simulink library "sadc_library_old"  (R2020b)
settings: Solver=VariableStepAuto  StartTime=0.0  StopTime=10.0  RelTol=1e-3
undefined symbols (not defined in the file or in its folder): magnitude
libraries: vrlib x4
settings Model: Creator=loren  LastModifiedBy=loren

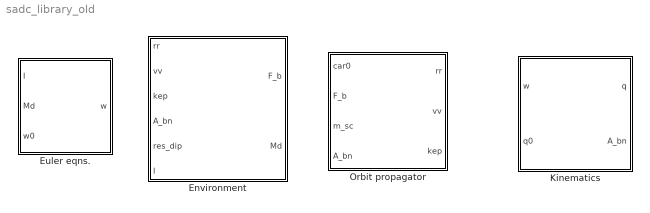
== system sadc_library_old ==
  Environment : Subsystem
  Euler eqns. : Subsystem
  Kinematics : Subsystem
  Orbit propagator : Subsystem

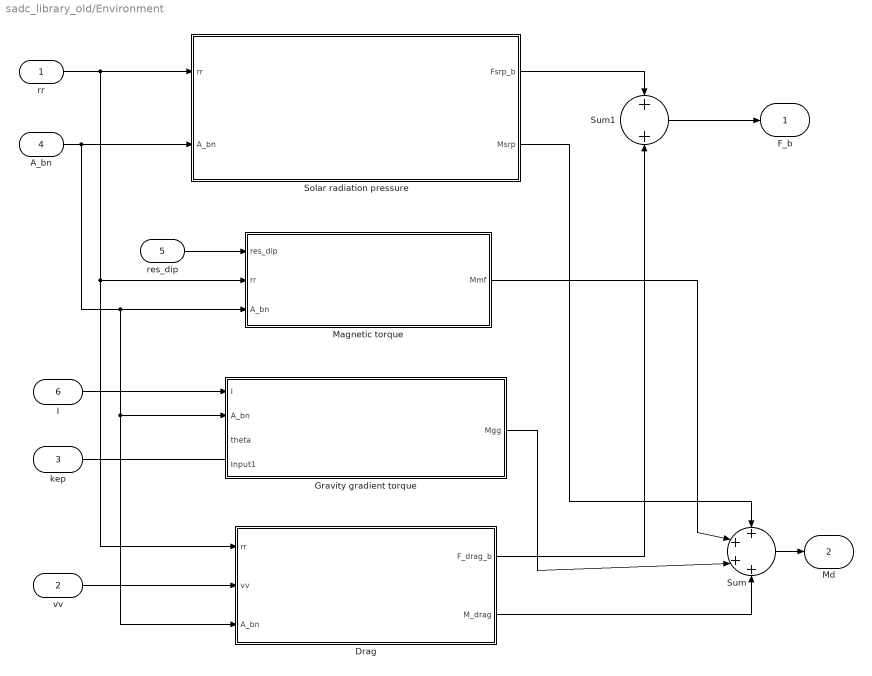
== system sadc_library_old/Environment ==
  rr : Inport
  vv : Inport  Port=2
  kep : Inport  Port=3
  A_bn : Inport  Port=4
  res_dip : Inport  Port=5
  I : Inport  Port=6
  Drag : Subsystem
  Gravity gradient torque : Subsystem
  Magnetic torque : Subsystem
  Solar radiation pressure : Subsystem
  Sum : Sum  Inputs=++++
  Sum1 : Sum
  F_b : Outport
  Md : Outport  Port=2
  wires:
  kep/1 -> ?
  Solar radiation pressure/1(Fsrp_b) -> Sum1/1
  Solar radiation pressure/2(Msrp) -> Sum/1
  A_bn/1 -> Drag/3(A_bn), Gravity gradient torque/2(A_bn), Magnetic torque/3(A_bn), Solar radiation pressure/2(A_bn)
  vv/1 -> Drag/2(vv)
  rr/1 -> Magnetic torque/2(rr), Drag/1(rr), Solar radiation pressure/1(rr)
  Gravity gradient torque/1(Mgg) -> Sum/3
  Drag/2(M_drag) -> Sum/4
  Drag/1(F_drag_b) -> Sum1/2
  I/1 -> Gravity gradient torque/1(I)
  res_dip/1 -> Magnetic torque/1(res_dip)
  Magnetic torque/1(Mmf) -> Sum/2
  Sum1/1 -> F_b/1
  Sum/1 -> Md/1

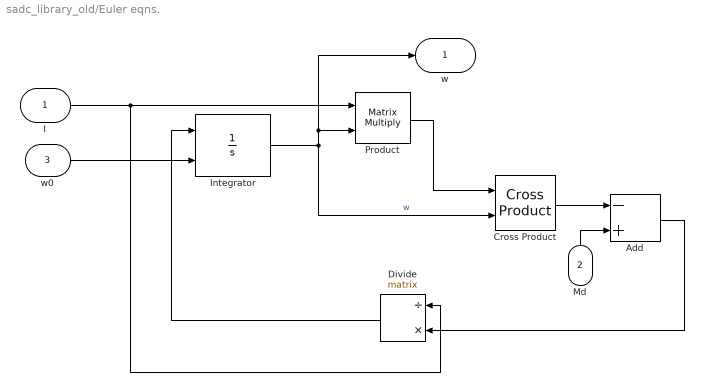
== system sadc_library_old/Euler eqns. ==
  I : Inport
  Md : Inport  Port=2
  w0 : Inport  Port=3
  Add : Sum  Inputs=-+
  Cross Product : vrlib/Utilities/Cross Product
  Divide : Product  Inputs=/*  Multiplication=Matrix(*)
  Integrator : Integrator  InitialConditionSource=external
  Product : Product  Multiplication=Matrix(*)
  w : Outport
  wires:
  I/1 -> Divide/1, Product/1
  w0/1 -> Integrator/2
  Integrator/1 -> Product/2, w/1, Cross Product/2  "w"
  Product/1 -> Cross Product/1
  Md/1 -> Add/2
  Cross Product/1 -> Add/1
  Add/1 -> Divide/2
  Divide/1 -> Integrator/1

== system sadc_library_old/Kinematics ==
  w : Inport
  q0 : Inport  Port=2
  DCM : Subsystem
  Quaternion integration : Subsystem
  q : Outport
  A_bn : Outport  Port=2
  wires:
  w/1 -> Quaternion integration/1(w)
  q0/1 -> Quaternion integration/2(q0)
  Quaternion integration/1(q) -> q/1, DCM/1(q)
  DCM/1(A_bn) -> A_bn/1

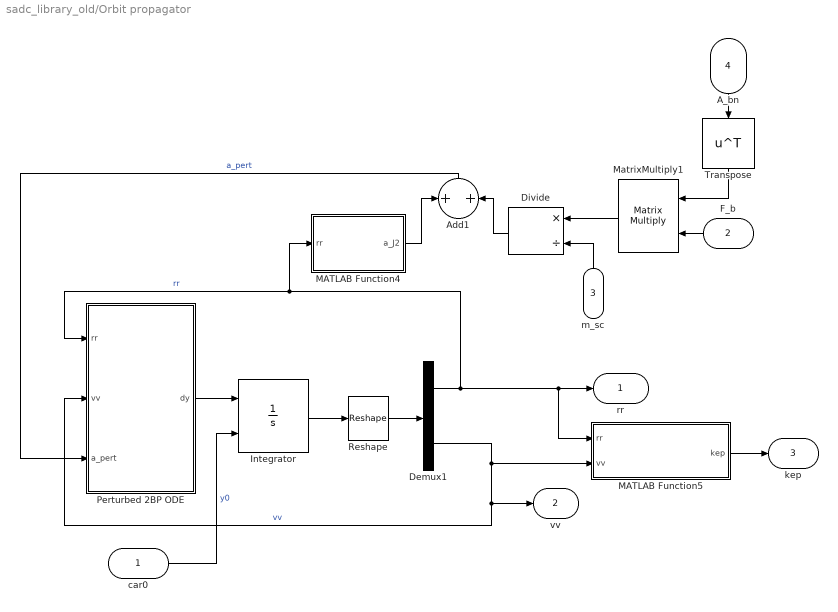
== system sadc_library_old/Orbit propagator ==
  car0 : Inport
  F_b : Inport  Port=2
  m_sc : Inport  Port=3
  A_bn : Inport  Port=4
  Add1 : Sum
  Demux1 : Demux  Outputs=[3,3]
  Divide : Product  Inputs=*/
  Integrator : Integrator  InitialConditionSource=external
  MATLAB Function4 : MATLAB Function  TreatAsAtomicUnit=on
  MATLAB Function5 : MATLAB Function  TreatAsAtomicUnit=on
  MatrixMultiply1 : Product  Multiplication=Matrix(*)
  Perturbed 2BP ODE : Subsystem
  Reshape : Reshape  OutputDimensionality=Column vector (2-D)
  Transpose : Math  Operator=transpose  SaturateOnIntegerOverflow=on
  rr : Outport
  vv : Outport  Port=2
  kep : Outport  Port=3
  wires:
  Integrator/1 -> Reshape/1
  Demux1/1 -> MATLAB Function5/1(rr), rr/1, MATLAB Function4/1(rr), Perturbed 2BP ODE/1(rr)  "rr"
  Perturbed 2BP ODE/1(dy) -> Integrator/1
  Demux1/2 -> vv/1, Perturbed 2BP ODE/2(vv), MATLAB Function5/2(vv)  "vv"
  car0/1 -> Integrator/2  "y0"
  Add1/1 -> Perturbed 2BP ODE/3(a_pert)  "a_pert"
  MATLAB Function4/1(a_J2) -> Add1/1
  F_b/1 -> MatrixMultiply1/2
  MatrixMultiply1/1 -> Divide/1
  m_sc/1 -> Divide/2
  Divide/1 -> Add1/2
  MATLAB Function5/1(kep) -> kep/1
  A_bn/1 -> Transpose/1
  Transpose/1 -> MatrixMultiply1/1
  Reshape/1 -> Demux1/1

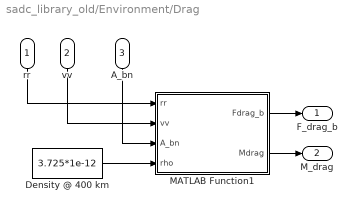
== system sadc_library_old/Environment/Drag ==
  rr : Inport
  vv : Inport  Port=2
  A_bn : Inport  Port=3
  Density @ 400 km : Constant  Value=3.725*1e-12
  MATLAB Function1 : MATLAB Function  TreatAsAtomicUnit=on
  F_drag_b : Outport
  M_drag : Outport  Port=2
  wires:
  rr/1 -> MATLAB Function1/1(rr)
  MATLAB Function1/1(Fdrag_b) -> F_drag_b/1
  MATLAB Function1/2(Mdrag) -> M_drag/1
  vv/1 -> MATLAB Function1/2(vv)
  A_bn/1 -> MATLAB Function1/3(A_bn)
  Density @ 400 km/1 -> MATLAB Function1/4(rho)

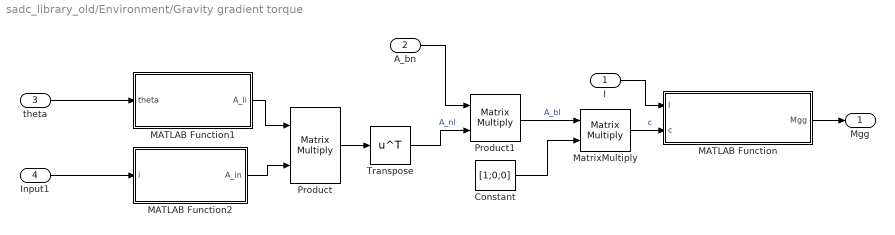
== system sadc_library_old/Environment/Gravity gradient torque ==
  I : Inport
  A_bn : Inport  Port=2
  theta : Inport  Port=3
  Input1 : Inport  Port=4
  Constant : Constant  Value=[1;0;0]
  MATLAB Function : MATLAB Function  TreatAsAtomicUnit=on
  MATLAB Function1 : MATLAB Function  TreatAsAtomicUnit=on
  MATLAB Function2 : MATLAB Function  TreatAsAtomicUnit=on
  MatrixMultiply : Product  Multiplication=Matrix(*)
  Product : Product  Multiplication=Matrix(*)
  Product1 : Product  Multiplication=Matrix(*)
  Transpose : Math  Operator=transpose  SaturateOnIntegerOverflow=on
  Mgg : Outport
  wires:
  I/1 -> MATLAB Function/1(I)
  Product/1 -> Transpose/1
  Transpose/1 -> Product1/2  "A_nl"
  Product1/1 -> MatrixMultiply/1  "A_bl"
  A_bn/1 -> Product1/1
  Constant/1 -> MatrixMultiply/2
  MatrixMultiply/1 -> MATLAB Function/2(c)  "c"
  MATLAB Function/1(Mgg) -> Mgg/1
  MATLAB Function2/1(A_in) -> Product/2
  MATLAB Function1/1(A_li) -> Product/1
  theta/1 -> MATLAB Function1/1(theta)
  Input1/1 -> MATLAB Function2/1(i)

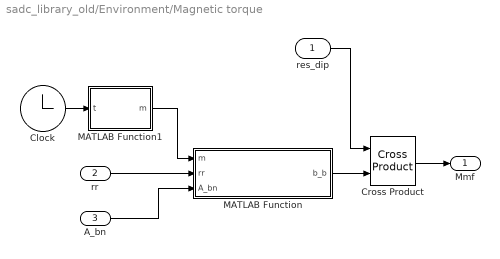
== system sadc_library_old/Environment/Magnetic torque ==
  res_dip : Inport
  rr : Inport  Port=2
  A_bn : Inport  Port=3
  Clock : Clock
  Cross Product : vrlib/Utilities/Cross Product
  MATLAB Function : MATLAB Function  TreatAsAtomicUnit=on
  MATLAB Function1 : MATLAB Function  TreatAsAtomicUnit=on
  Mmf : Outport
  wires:
  Cross Product/1 -> Mmf/1
  Clock/1 -> MATLAB Function1/1(t)
  rr/1 -> MATLAB Function/2(rr)
  A_bn/1 -> MATLAB Function/3(A_bn)
  res_dip/1 -> Cross Product/1
  MATLAB Function/1(b_b) -> Cross Product/2
  MATLAB Function1/1(m) -> MATLAB Function/1(m)

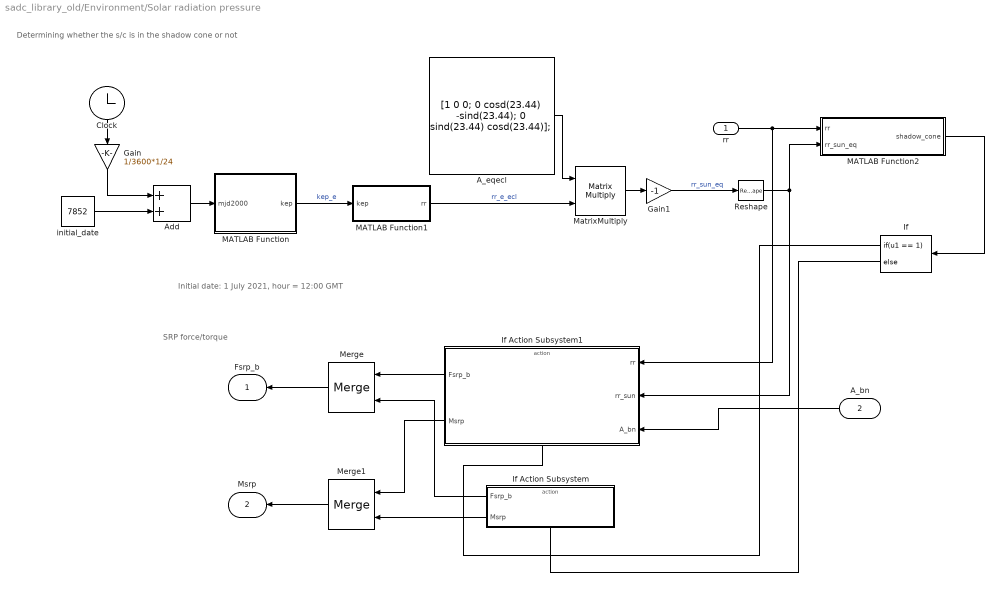
== system sadc_library_old/Environment/Solar radiation pressure ==
  note: SRP force/torque
  note: Initial date: 1 July 2021,
      | hour = 12:00 GMT
  note: Determining whether the s/c is in the shadow cone or not
  rr : Inport
  A_bn : Inport  Port=2
  A_eqecl : Constant  Value=|
      | [1   0   0;
      |     0  cosd(23.44)  -sind(23.44);
      |     0  sind(23.44)  cosd(23.44)];
  Add : Sum
  Clock : Clock
  Gain : Gain  Gain=1/3600*1/24
  Gain1 : Gain  Gain=-1
  If : If  IfExpression=u1 == 1
  If Action Subsystem : Subsystem  TreatAsAtomicUnit=on
  If Action Subsystem1 : Subsystem  TreatAsAtomicUnit=on
  MATLAB Function : MATLAB Function  TreatAsAtomicUnit=on
  MATLAB Function1 : MATLAB Function  TreatAsAtomicUnit=on
  MATLAB Function2 : MATLAB Function  TreatAsAtomicUnit=on
  MatrixMultiply : Product  Multiplication=Matrix(*)
  Merge : Merge
  Merge1 : Merge
  Reshape : Reshape  OutputDimensionality=Column vector (2-D)
  initial_date : Constant  Value=7852
  Fsrp_b : Outport
  Msrp : Outport  Port=2
  wires:
  initial_date/1 -> Add/2
  Clock/1 -> Gain/1
  Add/1 -> MATLAB Function/1(mjd2000)
  Gain/1 -> Add/1
  MatrixMultiply/1 -> Gain1/1
  MATLAB Function1/1(rr) -> MatrixMultiply/2  "rr_e_ecl"
  MATLAB Function/1(kep) -> MATLAB Function1/1(kep)  "kep_e"
  Gain1/1 -> Reshape/1  "rr_sun_eq"
  MATLAB Function2/1(shadow_cone) -> If/1
  If/2 -> If Action Subsystem/Action
  If/1 -> If Action Subsystem1/Action
  If Action Subsystem/1(Fsrp_b) -> Merge/2
  If Action Subsystem/2(Msrp) -> Merge1/2
  rr/1 -> MATLAB Function2/1(rr), If Action Subsystem1/1(rr)
  Merge/1 -> Fsrp_b/1
  Merge1/1 -> Msrp/1
  If Action Subsystem1/1(Fsrp_b) -> Merge/1
  If Action Subsystem1/2(Msrp) -> Merge1/1
  A_bn/1 -> If Action Subsystem1/3(A_bn)
  A_eqecl/1 -> MatrixMultiply/1
  Reshape/1 -> MATLAB Function2/2(rr_sun_eq), If Action Subsystem1/2(rr_sun)

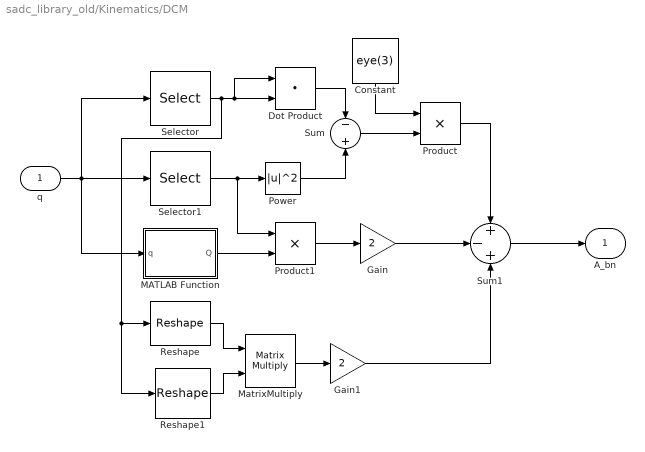
== system sadc_library_old/Kinematics/DCM ==
  q : Inport
  Constant : Constant  Value=eye(3)
  Dot Product : DotProduct  InputSameDT=on  OutDataTypeStr=Inherit: Inherit via internal rule
  Gain : Gain  Gain=2
  Gain1 : Gain  Gain=2
  MATLAB Function : MATLAB Function  TreatAsAtomicUnit=on
  MatrixMultiply : Product  Multiplication=Matrix(*)
  Power : Math  Operator=magnitude^2  SaturateOnIntegerOverflow=on
  Product : Product
  Product1 : Product
  Reshape : Reshape  OutputDimensionality=Column vector (2-D)
  Reshape1 : Reshape  OutputDimensionality=Row vector (2-D)
  Selector : Selector  InputPortWidth=4  IndexOptions=Index vector (dialog)  Indices=[1 2 3]  OutputSizes=1
  Selector1 : Selector  InputPortWidth=4  IndexOptions=Index vector (dialog)  Indices=[4]  OutputSizes=1
  Sum : Sum  Inputs=-+
  Sum1 : Sum  Inputs=+-+
  A_bn : Outport
  wires:
  q/1 -> MATLAB Function/1(q), Selector1/1, Selector/1
  Selector/1 -> Reshape1/1, Reshape/1, Dot Product/2, Dot Product/1
  Selector1/1 -> Product1/1, Power/1
  Power/1 -> Sum/2
  Dot Product/1 -> Sum/1
  Constant/1 -> Product/1
  Sum/1 -> Product/2
  MATLAB Function/1(Q) -> Product1/2
  Product1/1 -> Gain/1
  Reshape/1 -> MatrixMultiply/1
  Reshape1/1 -> MatrixMultiply/2
  MatrixMultiply/1 -> Gain1/1
  Product/1 -> Sum1/1
  Gain/1 -> Sum1/2
  Gain1/1 -> Sum1/3
  Sum1/1 -> A_bn/1

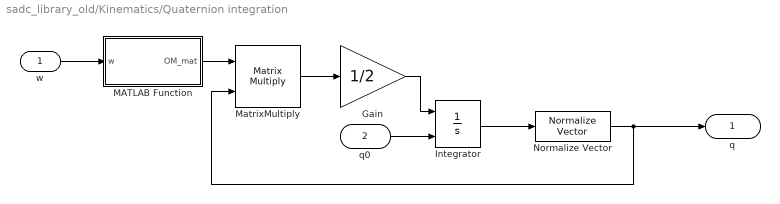
== system sadc_library_old/Kinematics/Quaternion integration ==
  w : Inport
  q0 : Inport  Port=2
  Gain : Gain  Gain=1/2
  Integrator : Integrator  InitialConditionSource=external
  MATLAB Function : MATLAB Function  TreatAsAtomicUnit=on
  MatrixMultiply : Product  Multiplication=Matrix(*)
  Normalize Vector : vrlib/Utilities/Normalize Vector  maxzero=0
  q : Outport
  wires:
  Integrator/1 -> Normalize Vector/1
  w/1 -> MATLAB Function/1(w)
  Normalize Vector/1 -> q/1, MatrixMultiply/2
  q0/1 -> Integrator/2
  MATLAB Function/1(OM_mat) -> MatrixMultiply/1
  MatrixMultiply/1 -> Gain/1
  Gain/1 -> Integrator/1

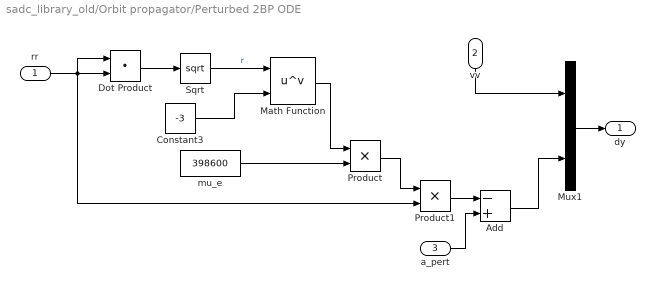
== system sadc_library_old/Orbit propagator/Perturbed 2BP ODE ==
  rr : Inport
  vv : Inport  Port=2
  a_pert : Inport  Port=3
  Add : Sum  Inputs=-+
  Constant3 : Constant  Value=-3
  Dot Product : DotProduct  InputSameDT=on  OutDataTypeStr=Inherit: Inherit via internal rule
  Math Function : Math  Operator=pow  SaturateOnIntegerOverflow=on
  Mux1 : Mux  Inputs=[3,3]
  Product : Product
  Product1 : Product
  Sqrt : Sqrt  SaturateOnIntegerOverflow=on
  mu_e : Constant  Value=398600
  dy : Outport
  wires:
  rr/1 -> Dot Product/1, Product1/2, Dot Product/2
  Add/1 -> Mux1/2
  Math Function/1 -> Product/1
  Mux1/1 -> dy/1
  Dot Product/1 -> Sqrt/1
  Product1/1 -> Add/1
  Product/1 -> Product1/1
  Constant3/1 -> Math Function/2
  a_pert/1 -> Add/2
  Sqrt/1 -> Math Function/1  "r"
  vv/1 -> Mux1/1
  mu_e/1 -> Product/2

== system sadc_library_old/Environment/Solar radiation pressure/If Action Subsystem ==
  Action Port : ActionPort
  Constant : Constant  Value=[0;0;0]
  Constant1 : Constant  Value=[0;0;0]
  Fsrp_b : Outport
  Msrp : Outport  Port=2
  wires:
  Constant/1 -> Fsrp_b/1
  Constant1/1 -> Msrp/1

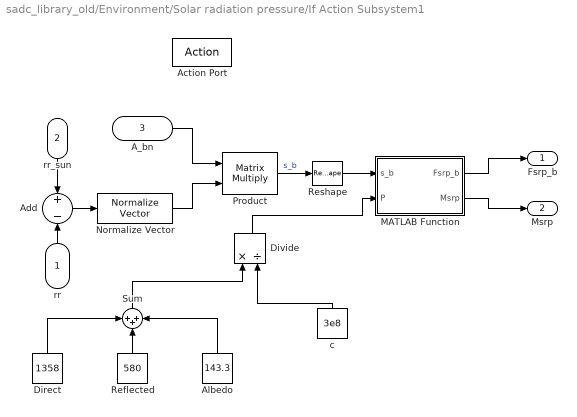
== system sadc_library_old/Environment/Solar radiation pressure/If Action Subsystem1 ==
  rr : Inport
  rr_sun : Inport  Port=2
  A_bn : Inport  Port=3
  Action Port : ActionPort
  Add : Sum  Inputs=+-
  Albedo : Constant  Value=143.3
  Direct : Constant  Value=1358
  Divide : Product  Inputs=*/
  MATLAB Function : MATLAB Function  TreatAsAtomicUnit=on
  Normalize Vector : vrlib/Utilities/Normalize Vector  maxzero=0
  Product : Product  Multiplication=Matrix(*)
  Reflected : Constant  Value=580
  Reshape : Reshape  OutputDimensionality=Column vector (2-D)
  Sum : Sum  Inputs=+++
  c : Constant  Value=3e8
  Fsrp_b : Outport
  Msrp : Outport  Port=2
  wires:
  A_bn/1 -> Product/1
  rr_sun/1 -> Add/1
  Product/1 -> Reshape/1  "s_b"
  Normalize Vector/1 -> Product/2
  Add/1 -> Normalize Vector/1
  MATLAB Function/1(Fsrp_b) -> Fsrp_b/1
  MATLAB Function/2(Msrp) -> Msrp/1
  Reflected/1 -> Sum/2
  Albedo/1 -> Sum/3
  Direct/1 -> Sum/1
  Sum/1 -> Divide/1
  c/1 -> Divide/2
  Divide/1 -> MATLAB Function/2(P)
  rr/1 -> Add/2
  Reshape/1 -> MATLAB Function/1(s_b)

== matlab function sadc_library_old/Environment/Gravity gradient torque/MATLAB Function2 ==
  data: i input; A_in output
function A_in = inertial_to_inclined(i)

A_in = [1, 0, 0;...
    0, cos(i), sin(i);...
    0, -sin(i), cos(i)];

end

== matlab function sadc_library_old/Environment/Drag/MATLAB Function1 ==
  data: rr input; vv input; A_bn input; rho input; Fdrag_b output; Mdrag output; surfaces parameter
function [Fdrag_b, Mdrag] = drag(rr, vv, A_bn, rho, surfaces)

we_vec = [0; 0; 7.2921150e-5];
cd = surfaces.cd;

r_surf_body = surfaces.body.r_surf;
r_surf_panels = surfaces.panels.r_surf;

n_body = surfaces.body.n;
n_panels = surfaces.panels.n;

A_body = surfaces.body.A;
A_panels = surfaces.panels.A;

nf_body = size(r_surf_body,1);
nf_panels = size(r_surf_panels,1);

vv_atm = cross(we_vec,rr*1e3); % [m/s]
vv_rel = vv*1e3 - vv_atm; % Relative velocity in inertial frame [m/s]
v_rel = norm(vv_rel);
vv_b = A_bn*vv_rel;
v_b = norm(vv_b);
v_vec = vv_b/v_b;

c = -1/2*rho*cd*v_rel^2.*v_vec;

Fdrag_b = zeros(3,1);
Mdrag = zeros(3,1);

for k = 1:nf_panels
        n_dot = dot(n_panels(k,:), v_vec);
    if n_dot > 0
        A_cross = A_panels(k)*n_dot;
        Fdrag_i = c*A_cross;
        Fdrag_b = Fdrag_b + Fdrag_i;
        Mdrag = Mdrag + cross(r_surf_panels(k,:)', Fdrag_b);
    end
end

for k = 1:nf_body
    n_dot = dot(n_body(k,:), v_vec);
    if n_dot > 0
        A_cross = A_body(k)*n_dot;
        Fdrag_i = c*A_cross;
        Fdrag_b = Fdrag_b + Fdrag_i;
        Mdrag = Mdrag + cross(r_surf_body(k,:)', Fdrag_b);
    end
end


% aggiungere questione su "ombra aerodinamica"
end

== matlab function sadc_library_old/Kinematics/DCM/MATLAB Function ==
  data: q input; Q output
function Q = skew_matrix(q)

q1 = q(1);
q2 = q(2);
q3 = q(3);

Q = [0, -q3, q2;...
    q3, 0, -q1;...
    -q2, q1, 0];

end

== matlab function sadc_library_old/Environment/Magnetic torque/MATLAB Function1 ==
  data: m output; t input
function m = m_vector(t)

we = 7.2921150e-5;
m = [sind(11.5)*cos(we*t);...
    sind(11.5)*sin(we*t);...
    cosd(11.5)];

end

== matlab function sadc_library_old/Environment/Magnetic torque/MATLAB Function ==
  data: m input; rr input; b_b output; A_bn input
function b_b = magnetic_dipole(m, rr, A_bn)

H0 = 3.009279157871533e-05;
Req = 6378.1*1e3;
r_norm = norm(rr);
r_vec = rr/norm(rr)*1e3;

b_n = Req^3*H0/(r_norm^3)*(3*dot(m,r_vec)*r_vec - m);

b_b = A_bn*b_n;

end

== matlab function sadc_library_old/Environment/Gravity gradient torque/MATLAB Function ==
  data: Mgg output; I input; c input
function Mgg = gravity_gradient(I, c)

G = 6.67408e-11;
me = 5.97237e24;
Req = 6371.8e3;

c1 = c(1);
c2 = c(2);
c3 = c(3);
Ix = I(1,1);
Iy = I(2,2);
Iz = I(3,3);

Mgg = 3*G*me/(Req^3)*[(Iz - Iy)*c2*c3;...
    (Ix - Iz)*c1*c3;...
    (Iy - Ix)*c1*c2];

end

== matlab function sadc_library_old/Environment/Solar radiation pressure/MATLAB Function ==
  data: mjd2000 input; kep output
function  kep = uplanet(mjd2000)

% uplanet.m - Analytical ephemerides for planets
%
% PROTOTYPE:
%  [kep, ksun] = uplanet (mjd2000, ibody);
%
% DESCRIPTION:
%   Planetary orbital elements are restituited in a Sun-centred ecliptic 
%   system.
%   These ephemerides were succesfully compared with JPL/NAIF/SPICE
%   ephemerides using de405.bps.
%
%  INPUT :
%	mjd2000[1]  Time, modified Julian day since 01/01/2000, 12:00 noon
%               (MJD2000 = MJD-51544.5)
%	ibody[1]    Integer number identifying the celestial body (< 11)
%                   1:   Mercury
%                   2:   Venus
%                   3:   Earth
%                   4:   Mars
%                   5:   Jupiter
%                   6:   Saturn
%                   7:   Uranus
%                   8:   Neptune
%                   9:   Pluto
%                   10:  Sun
%
%  OUTPUT:
%	kep[6]    	Mean Keplerian elements of date
%                 kep = [a e i Om om theta] [km, rad]
%	ksun[1]     Gravity constant of the Sun [km^3/s^2]
%
%   Note: The ephemerides of the Moon are given by EphSS_kep, according to
%           to the algorithm in ephMoon.m
%
%  FUNCTIONS CALLED:
%   (none)
%
% AUTHOR:
%   P. Dysli, 1977
%
% PREVIOUS VERSION:
%   P. Dysli, 1977, MATLAB, uplanet.m
%       - Header and function name in accordance with guidlines.
%
%  CHANGELOG:
%   28/12/06, Camilla Colombo: tidied up
%   10/01/2007, REVISION, Matteo Ceriotti 
%   03/05/2008, Camilla Colombo: Case 11 deleted.
%   11/09/2008, Matteo Ceriotti, Camilla Colombo:
%       - All ephemerides shifted 0.5 days back in time. Now mjd2000 used
%           in this function is referred to 01/01/2000 12:00. In the old
%           version it was referred to 02/01/2000 00:00.
%       - Corrected ephemeris of Pluto.
%   04/10/2010, Camilla Colombo: Header and function name in accordance
%       with guidlines.
%
% -------------------------------------------------------------------------

DEG2RAD=pi/180;

G=6.67259e-20;
msun=1.988919445342813e+030;
kep = zeros(6,1);
KM  = 149597870.66;

%  T = JULIAN CENTURIES SINCE 31/12/1899 at 12:00
T   = (mjd2000 + 36525)/36525.00;
TT  = T*T;
TTT = T*TT;
kep(1)=T*0;

%
%  CLASSICAL PLANETARY ELEMENTS ESTIMATION IN MEAN ECLIPTIC OF DATE
%

    %  EARTH
    %
        kep(1) = 1.000000230;
        kep(2) = 0.016751040 - 0.000041800*T - 0.0000001260*TT;
        kep(3) = 0.00;
    	kep(4) = 0.00;
      	kep(5) = 1.01220833333333333e+2 + 1.7191750*T + 4.52777777777777778e-4*TT + 3.33333333333333333e-6*TTT;
     	XM   = 3.599904975e+4 - 1.50277777777777778e-4*T - 3.33333333333333333e-6*TT;
     	kep(6) = 3.58475844444444444e2 + XM*T;

  
%
%  CONVERSION OF AU INTO KM, DEG INTO RAD AND DEFINITION OF  XMU
%
 
kep(1)   = kep(1)*KM;       % a [km]
kep(3:6) = kep(3:6)*DEG2RAD;    % Transform from deg to rad
kep(6)   = mod(kep(6),2*pi);
% XMU  = (XM*DEG2RAD/(864000*365250))^2*kep(1)^3;
phi    = kep(6);          % phi is the eccentric anomaly, uses kep(6)=M as a first guess
     
for i=1:5
    g       = kep(6)-(phi-kep(2)*sin(phi)); 
	g_primo = (-1+kep(2)*cos(phi));
 	phi     = phi-g/g_primo;   % Computes the eccentric anomaly kep
end 

theta=2*atan(sqrt((1+kep(2))/(1-kep(2)))*tan(phi/2));

kep(6)=theta;

return

== matlab function sadc_library_old/Environment/Solar radiation pressure/MATLAB Function1 ==
  data: kep input; rr output
function rr = kep2car(kep)
% 
% Function to compute position and velocity vectors of the satellite the 
% keplerian elements.
% 
% INPUT:
%  a [1]       Semimajor axis [km]
%  e [1]       Eccentricity [-]
%  i [1]       Inclination angle [rad]
%  OM [1]      Right ascention of the ascending node [rad]
%  om [1]      Anomaly of the pericenter [rad]
%  th [1]      True anomaly [rad]
%  MU [1]      Gravitational parameter of the primary [km^3/s^2]
% 
% OUTPUT:
%  rr [3,1]    Position vector in inertial frame [km]
%  vv [3,1]    Velocity vector in inertial frame [km/s]
% 
a = kep(1); e = kep(2); i = kep(3); OM = kep(4); om = kep(5); theta = kep(6);

p = a*(1-e^2);
r = p/(1+e*cos(theta));

rr = r*[cos(theta);sin(theta);0];

ROM = [ cos(OM) sin(OM) 0; -sin(OM) cos(OM) 0; 0 0 1];
Ri = [ 1 0 0; 0 cos(i) sin(i); 0 -sin(i) cos(i)];
Rom = [ cos(om) sin(om) 0; -sin(om) cos(om) 0; 0 0 1];

T = Rom*Ri*ROM;

rr = T'*rr;

end

== matlab function sadc_library_old/Environment/Solar radiation pressure/MATLAB Function2 ==
  data: rr input; shadow_cone output; rr_sun_eq input
function shadow_cone = cone(rr, rr_sun_eq)

% PROTOTYPE:
%  shadow_cone = cone(rr_sc, rr_sun)
% 
% DESCRIPTION:
%   This function returns a parameter that is 1 if the s/c is out of the 
%   planet's shadow cone (SRP effects considerable) or 0 if the s/c is 
%   inside the planet's shadow cone (NO SRP)
% 
% INPUT:
% rr_sc:            geocentric position vector of the s/c
% rr_sun_eq:        geocentric position vector of the sun
%
% OUTPUT:
% shadow_cone:      boolean parameter (0 or 1)
%
% CONTRIBUTORS:
% Velo Giacomo
%
% VERSIONS:
% 2019-12-10 first version
%
% CALLED FUNCTIONS:
%     none


R_e = 6378.137;
r_sc = norm(rr);     
r_sun = norm(rr_sun_eq);
% Angle between s/c geocentric position and the tangent to Earth's surface
theta_sc = acos(R_e/r_sc);
% Angle between sun geocentric position and the tangent to Earth's surface
theta_sun = acos(R_e/r_sun);
% Angle between s/c geocentric position and sun geocentric position
theta = acos(dot(rr, rr_sun_eq)/(r_sc*r_sun));

% If the s/c is inside the shadow cone of the planet the value of
% shadow_cone will be = 0

    if theta_sc + theta_sun <= theta
        shadow_cone = 0;
    else
        shadow_cone = 1;
    end

end

== matlab function sadc_library_old/Kinematics/Quaternion integration/MATLAB Function ==
  data: w input; OM_mat output
function OM_mat = quat_matrix(w)

wx = w(1);
wy = w(2);
wz = w(3);

OM_mat = [0, wz, -wy, wx;...
    -wx, 0, wx, wy;...
    wy, -wx, 0, wz;...
    -wx, -wy, -wz, 0];
    
end

== matlab function sadc_library_old/Orbit propagator/MATLAB Function4 ==
  data: a_J2 output; rr input
function a_J2 = J2_perturb(rr)

J2 = 0.00108263;
Req = 6378.1;
mu_e = 398600;

r = norm(rr);
rx = rr(1);
ry = rr(2);
rz = rr(3);

a_J2 = 3/2*J2*mu_e*Req^2/(r^4)*[rx/r*(5*(rz/r)^2 - 1);...
    ry/r*(5*(rz/r)^2 - 1);...
    rz/r*(5*(rz/r)^2 - 3)];

end

== matlab function sadc_library_old/Orbit propagator/MATLAB Function5 ==
  data: rr input; kep output; vv input
function kep = car2kep(rr, vv)

mu_e = 398600;

r = norm(rr);
v = norm(vv);

hh = cross(rr,vv);
h = norm(hh);
i = acos(hh(3)/h);

a = -mu_e/2*1/(v^2/2 - mu_e/r);

k = [0 0 1];
nn = cross(k,hh);
nn = nn/norm(nn);

if nn(2) < 0
    OM = 2*pi - acos(nn(1));
else
    OM = acos(nn(1));
end

ee = cross(vv,hh)/mu_e - rr/r;
e = norm(ee);

if ee(3) < 0
    om = 2*pi - acos(dot(nn,ee)/e);
else
    om = acos(dot(nn,ee)/e);
end

vr = dot(rr,vv);

if vr < 0
    theta = 2*pi - acos(dot(rr,ee)/r/e);
else
    theta = acos(dot(rr,ee)/r/e);
end

kep = [a; e; i; OM; om; theta];

end

== matlab function sadc_library_old/Environment/Solar radiation pressure/If Action Subsystem1/MATLAB Function ==
  data: s_b input; P input; Fsrp_b output; Msrp output; surfaces parameter
function [Fsrp_b, Msrp] = srp(s_b, P, surfaces)

rhoS_body = surfaces.body.rhoS;
rhoD_body = surfaces.body.rhoD;

rhoS_panels = surfaces.panels.rhoS;
rhoD_panels = surfaces.panels.rhoD;

nf_body = surfaces.body.num;
nf_panels = surfaces.panels.num;

r_surf_body = surfaces.body.r_surf;
r_surf_panels = surfaces.panels.r_surf;
n_body = surfaces.body.n;
n_panels = surfaces.panels.n;

A_body = surfaces.body.A;
A_panels = surfaces.panels.A;

Fsrp_b = zeros(3,1);
Msrp = zeros(3,1);

for k = 1:nf_panels
    n_b = n_panels(k,:)';
    s_dot = dot(s_b, n_b);
    if s_dot > 0
        Fsrp_i = - P*A_panels(k)*s_dot.*((1-rhoS_panels).*s_b +...
            (2*rhoS_panels*s_dot + 2/3*rhoD_panels).*n_b);
        Fsrp_b = Fsrp_b + Fsrp_i;
        Msrp = Msrp + cross(r_surf_panels(k,:)', Fsrp_i);
    end
end

for k = 1:nf_body
    n_b = n_body(k,:)';
    s_dot = dot(s_b, n_b);
    if s_dot > 0
        Fsrp_i = - P*A_body(k)*s_dot.*((1-rhoS_body).*s_b +...
            (2*rhoS_body*s_dot + 2/3*rhoD_body).*n_b);
        Fsrp_b = Fsrp_b + Fsrp_i;
        Msrp = Msrp + cross(r_surf_body(k,:)', Fsrp_i);
    end
end

% aggiungere questione su "ombra aerodinamica"

end

== matlab function sadc_library_old/Environment/Gravity gradient torque/MATLAB Function1 ==
  data: theta input; A_li output
function A_li = inclined_to_orbital(theta)

A_li = [cos(theta), sin(theta), 0;...
    -sin(theta), cos(theta), 0;...
    0, 0, 1];

end
